simulink model "soac_unit_test"  (R2016b)
settings: Solver=FixedStepAuto  StartTime=0.0  StopTime=1  RelTol=1e-3
values from neighbouring files (symbols this model uses):
  hw0 = Jw * 0.10471975511966 * [ 1000; 1000; 1000 ]    [soac_unit_test_init.m]
  q0 = [ cosd(60/2); sind(60/2).*n ]    [soac_unit_test_init.m]
  qf = quatmultiply(qd',q0')'    [soac_unit_test_init.m]
  sI = [ 1.0; 0.0; 0.0 ]    [soac_unit_test_init.m]
  w0 = [ 0.0; 0.0; 0.0 ]    [soac_unit_test_init.m]
  wf = [ 0.0; 0.0; 0.0 ]    [soac_unit_test_init.m]
libraries: simulink x2, soac_lib x1
settings Model: Creator=Taylor  LastModifiedBy=Taylor
settings OptimizationCC: DefaultParameterBehavior=Inlined  UseDivisionForNetSlopeComputation=on  UseFloatMulNetSlope=on  InlineInvariantSignals=on  PassReuseOutputArgsAs=Individual arguments  ZeroExternalMemoryAtStartup=off  ZeroInternalMemoryAtStartup=off  NoFixptDivByZeroProtection=on  EfficientFloat2IntCast=on  LifeSpan=1
settings DebuggingCC: ParameterTunabilityLossMsg=error
settings HardwareCC: ProdBitPerPointer=32  ProdBitPerSizeT=32  ProdBitPerPtrDiffT=32  ProdLargestAtomicInteger=Long  ProdWordSize=32  ProdHWDeviceType=ARM Compatible->ARM 7
settings RTWCC: SystemTargetFile=ert.tlc  TemplateMakefile=ert_default_tmf  Description=Embedded Coder  GenerateReport=on  CustomInclude="\"/Users/Taylor/uw_cubesat_adcs/adcs/sw/components/adcs_oac/include/ecos/include\""  IncludeHyperlinkInReport=on  LaunchReport=on  GenerateTraceInfo=on  GenerateTraceReport=on  GenerateTraceReportSl=on  GenerateTraceReportSf=on  GenerateTraceReportEml=on  GenerateCodeMetricsReport=on
settings RTWCC: CustomSource=|
  | "/Users/Taylor/uw_cubesat_adcs/adcs/sw/components/adcs_oac/include/ecos/src/amd_1.c"
  | "/Users/Taylor/uw_cubesat_adcs/adcs/sw/components/adcs_oac/include/ecos/src/amd_2.c"
  | "/Users/Taylor/uw_cubesat_adcs/adcs/sw/components/adcs_oac/include/ecos/src/amd_aat.c"
  | "/Users/Taylor/uw_cubesat_adcs/adcs/sw/components/adcs_oac/include/ecos/src/amd_control.c"
  | "/Users/Taylor/uw_cubesat_adcs/adcs/sw/components/adcs_oac/include/ecos/src/amd_defaults.c"
  | "/Users/Taylor/uw_cubesat_adcs/adcs/sw/components/adcs_oac/include/ecos/src/amd_dump"
  | "/Users/Taylor/uw_cubesat_adcs/adcs/sw/components/adcs_oac/include/ecos/src/amd_global.c"
  | "/Users/Taylor/uw_cubesat_adcs/adcs/sw/components/adcs_oac/include/ecos/src/amd_info.c"
  | "/Users/Taylor/uw_cubesat_adcs/adcs/sw/components/adcs_oac/include/ecos/src/amd_order.c"
  | "/Users/Taylor/uw_cubesat_adcs/adcs/sw/components/adcs_oac/include/ecos/src/amd_post_tree.c"
  | "/Users/Taylor/uw_cubesat_adcs/adcs/sw/components/adcs_oac/include/ecos/src/amd_postorder.c"
  | "/Users/Taylor/uw_cubesat_adcs/adcs/sw/components/adcs_oac/include/ecos/src/amd_preprocess.c"
  | "/Users/Taylor/uw_cubesat_adcs/adcs/sw/components/adcs_oac/include/ecos/src/amd_valid.c"
  | "/Users/Taylor/uw_cubesat_adcs/adcs/sw/components/adcs_oac/include/ecos/src/cone.c"
  | "/Users/Taylor/uw_cubesat_adcs/adcs/sw/components/adcs_oac/include/ecos/src/ctrlc.c"
  | "/Users/Taylor/uw_cubesat_adcs/adcs/sw/components/adcs_oac/include/ecos/src/ecos.c"
  | "/Users/Taylor/uw_cubesat_adcs/adcs/sw/components/adcs_oac/include/ecos/src/equil.c"
  | "/Users/Taylor/uw_cubesat_adcs/adcs/sw/components/adcs_oac/include/ecos/src/expcone.c"
  | "/Users/Taylor/uw_cubesat_adcs/adcs/sw/components/adcs_oac/include/ecos/src/kkt.c"
  | "/Users/Taylor/uw_cubesat_adcs/adcs/sw/components/adcs_oac/include/ecos/src/ldl.c"
  | "/Users/Taylor/uw_cubesat_adcs/adcs/sw/components/adcs_oac/include/ecos/src/matlab_main.c"
  | "/Users/Taylor/uw_cubesat_adcs/adcs/sw/components/adcs_oac/include/ecos/src/preproc.c"
  | "/Users/Taylor/uw_cubesat_adcs/adcs/sw/components/adcs_oac/include/ecos/src/runecos.c"
  | "/Users/Taylor/uw_cubesat_adcs/adcs/sw/components/adcs_oac/include/ecos/src/spla.c"
  | "/Users/Taylor/uw_cubesat_adcs/adcs/sw/components/adcs_oac/include/ecos/src/splamm.c"
  | "/Users/Taylor/uw_cubesat_adcs/adcs/sw/components/adcs_oac/include/ecos/src/timer.c"
  | "/Users/Taylor/uw_cubesat_adcs/adcs/sw/components/adcs_oac/include/ecos/src/wright_omega.c"
settings CodeAppCC: ForceParamTrailComments=on  IgnoreCustomStorageClasses=off  OperatorAnnotations=on  SimulinkDataObjDesc=on  SFDataObjDesc=on  MATLABFcnDesc=on  CustomSymbolStrGlobalVar=rt$N$M  CustomSymbolStrType=$N$M  CustomSymbolStrFcn=$N$M$F  CustomSymbolStrMacro=$N$M  InsertBlockDesc=on  MATLABSourceComments=on
settings ERTTargetCC: TargetLangStandard=C99 (ISO)  GenerateSampleERTMain=on  CombineSignalStateStructs=on  SupportAbsoluteTime=off  SupportComplex=off  SupportContinuousTime=on  SupportNonInlinedSFcns=on  InlinedParameterPlacement=NonHierarchical  ERTCustomFileTemplate=example_file_process.tlc  ERTFilePackagingFormat=CompactWithDataFile

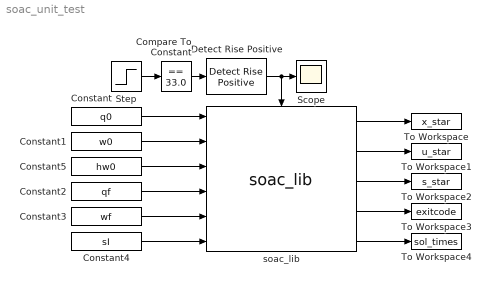
== system soac_unit_test ==
  Compare To Constant : simulink/Logic and Bit Operations/Compare To Constant  relop===  const=33.0  OutDataTypeStr=boolean
  Constant : Constant  Value=q0
  Constant1 : Constant  Value=w0
  Constant2 : Constant  Value=qf
  Constant3 : Constant  Value=wf
  Constant4 : Constant  Value=sI
  Constant5 : Constant  Value=hw0
  Detect Rise Positive : simulink/Logic and Bit Operations/Detect Rise Positive  vinit=0  OutDataTypeStr=boolean
  Scope : Scope
  Step : Step  Time=0  After=33  SampleTime=0
  To Workspace : ToWorkspace  VariableName=x_star  SampleTime=-1
  To Workspace1 : ToWorkspace  VariableName=u_star  SampleTime=-1
  To Workspace2 : ToWorkspace  VariableName=s_star  SampleTime=-1
  To Workspace3 : ToWorkspace  VariableName=exitcode  SampleTime=-1
  To Workspace4 : ToWorkspace  VariableName=sol_times  SampleTime=-1
  soac_lib : soac_lib/soac_lib
  wires:
  Constant/1 -> soac_lib/1
  Constant1/1 -> soac_lib/2
  Constant2/1 -> soac_lib/4
  Constant3/1 -> soac_lib/5
  Constant4/1 -> soac_lib/6
  soac_lib/1 -> To Workspace/1
  soac_lib/2 -> To Workspace1/1
  soac_lib/3 -> To Workspace2/1
  soac_lib/4 -> To Workspace3/1
  soac_lib/5 -> To Workspace4/1
  Step/1 -> Compare To Constant/1
  Compare To Constant/1 -> Detect Rise Positive/1
  Detect Rise Positive/1 -> soac_lib/Trigger, Scope/1
  Constant5/1 -> soac_lib/3
